simulink model "exosketon_robot_advanced_robotic"  (R2020b)
settings: Solver=FixedStepAuto  StartTime=0.0  StopTime=12  FixedStep=0.1  RelTol=1e-3
undefined symbols (not defined in the file): L_1, L_2, m_31, m_32
settings Model: Creator=A family  LastModifiedBy=A family

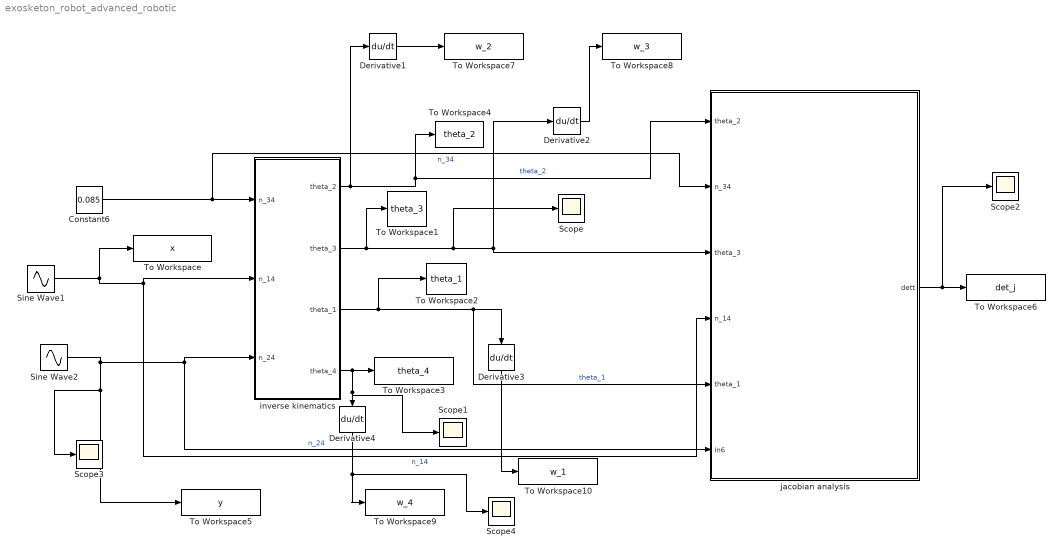
== system exosketon_robot_advanced_robotic ==
  Constant6 : Constant  Value=0.085
  Derivative{1..4} (4 alike) : Derivative
  Scope{,1..4} (5 alike) : Scope
  Sine Wave1 : Sin  Amplitude=0.2  Frequency=0.2  SampleTime=0
  Sine Wave2 : Sin  Amplitude=0.2  Frequency=0.2  Phase=-pi/2  SampleTime=0
  To Workspace : ToWorkspace  VariableName=x  SampleTime=-1
  To Workspace1 : ToWorkspace  VariableName=theta_3  SampleTime=-1
  To Workspace10 : ToWorkspace  VariableName=w_1  SampleTime=-1
  To Workspace2 : ToWorkspace  VariableName=theta_1  SampleTime=-1
  To Workspace3 : ToWorkspace  VariableName=theta_4  SampleTime=-1
  To Workspace4 : ToWorkspace  VariableName=theta_2  SampleTime=-1
  To Workspace5 : ToWorkspace  VariableName=y  SampleTime=-1
  To Workspace6 : ToWorkspace  VariableName=det_j  SampleTime=-1
  To Workspace7 : ToWorkspace  VariableName=w_2  SampleTime=-1
  To Workspace8 : ToWorkspace  VariableName=w_3  SampleTime=-1
  To Workspace9 : ToWorkspace  VariableName=w_4  SampleTime=-1
  inverse kinematics : Subsystem
  jacobian analysis : Subsystem
  wires:
  Constant6/1 -> jacobian analysis/2(n_34), inverse kinematics/1(n_34)  "n_34"
  Sine Wave1/1 -> inverse kinematics/2(n_14), jacobian analysis/4(n_14), To Workspace/1  "n_14"
  Sine Wave2/1 -> Scope3/1, To Workspace5/1, inverse kinematics/3(n_24), jacobian analysis/6(In6)  "n_24"
  inverse kinematics/4(theta_4) -> Scope1/1, Derivative4/1, To Workspace3/1
  inverse kinematics/3(theta_1) -> jacobian analysis/5(theta_1), Derivative3/1, To Workspace2/1  "theta_1"
  inverse kinematics/2(theta_3) -> Scope/1, Derivative2/1, jacobian analysis/3(theta_3), To Workspace1/1
  inverse kinematics/1(theta_2) -> Derivative1/1, To Workspace4/1, jacobian analysis/1(theta_2)  "theta_2"
  Derivative1/1 -> To Workspace7/1
  Derivative2/1 -> To Workspace8/1
  Derivative4/1 -> Scope4/1, To Workspace9/1
  Derivative3/1 -> To Workspace10/1
  jacobian analysis/1(dett) -> Scope2/1, To Workspace6/1

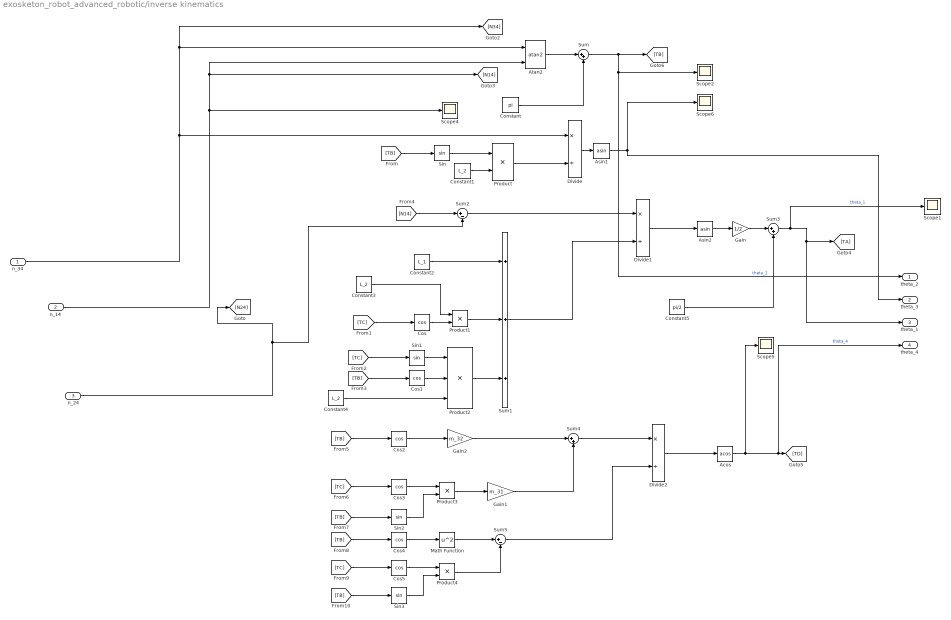
== system exosketon_robot_advanced_robotic/inverse kinematics ==
  n_34 : Inport
  n_14 : Inport  Port=2
  n_24 : Inport  Port=3
  Acos : Trigonometry  Operator=acos
  Asin1 : Trigonometry  Operator=asin
  Asin2 : Trigonometry  Operator=asin
  Atan2 : Trigonometry  Operator=atan2
  Constant : Constant  Value=pi
  Constant1 : Constant  Value=L_2
  Constant2 : Constant  Value=L_1
  Constant3 : Constant  Value=L_2
  Constant4 : Constant  Value=L_2
  Constant5 : Constant  Value=pi/2
  Cos{,1..5} (6 alike) : Trigonometry  Operator=cos
  Divide : Product  Inputs=*/
  Divide1 : Product  Inputs=*/
  Divide2 : Product  Inputs=*/
  Gain : Gain  Gain=1/2
  Gain1 : Gain  Gain=m_31
  Gain2 : Gain  Gain=m_32
  Math Function : Math  Operator=square  SaturateOnIntegerOverflow=on
  Product{,1,3..4} (4 alike) : Product
  Product2 : Product  Inputs=3
  Scope{1..2,4..6} (5 alike) : Scope
  Sin{,1..3} (4 alike) : Trigonometry
  Sum : Sum  Inputs=|++
  Sum1 : Sum  Inputs=+++
  Sum2 : Sum  Inputs=|+-
  Sum3 : Sum  Inputs=|++
  Sum4 : Sum  Inputs=|++
  Sum5 : Sum  Inputs=|+-
  theta_2 : Outport
  theta_3 : Outport  Port=2
  theta_1 : Outport  Port=3
  theta_4 : Outport  Port=4
  wires:
  Product2/1 -> Sum1/3
  Cos3/1 -> Product3/1
  Asin2/1 -> Gain/1
  Sum3/1 -> theta_1/1, [TA], Scope1/1  "theta_1"
  n_34/1 -> [N34], Atan2/1, Divide/1
  Constant1/1 -> Product/2
  Product3/1 -> Gain1/1
  Constant4/1 -> Product2/3
  Cos/1 -> Product1/2
  Asin1/1 -> theta_3/1, Scope6/1
  Constant/1 -> Sum/2
  Product/1 -> Divide/2
  Constant2/1 -> Sum1/1
  [TC] -> Cos/1
  [TB] -> Sin/1
  Sum2/1 -> Divide1/1
  Divide2/1 -> Acos/1
  [TB] -> Cos4/1
  Divide1/1 -> Asin2/1
  Product1/1 -> Sum1/2
  Sin3/1 -> Product4/2
  Constant5/1 -> Sum3/2
  Gain1/1 -> Sum4/2
  Sin/1 -> Product/1
  Sum/1 -> theta_2/1, Scope2/1, [TB]  "theta_2"
  n_24/1 -> Sum2/2, [N24]
  Atan2/1 -> Sum/1
  n_14/1 -> [N14], Atan2/2, Scope4/1
  Sin2/1 -> Product3/2
  [TB] -> Sin2/1
  [TB] -> Cos2/1
  Cos1/1 -> Product2/2
  Math Function/1 -> Sum5/1
  Sum1/1 -> Divide1/2
  Sum4/1 -> Divide2/1
  Sum5/1 -> Divide2/2
  Gain2/1 -> Sum4/1
  Divide/1 -> Asin1/1
  Gain/1 -> Sum3/1
  Cos2/1 -> Gain2/1
  [TB] -> Cos1/1
  Acos/1 -> theta_4/1, [TD], Scope5/1  "theta_4"
  Sin1/1 -> Product2/1
  [TC] -> Sin1/1
  Constant3/1 -> Product1/1
  [TC] -> Cos5/1
  Cos4/1 -> Math Function/1
  [TB] -> Sin3/1
  Cos5/1 -> Product4/1
  Product4/1 -> Sum5/2
  [TC] -> Cos3/1
  [N14] -> Sum2/1

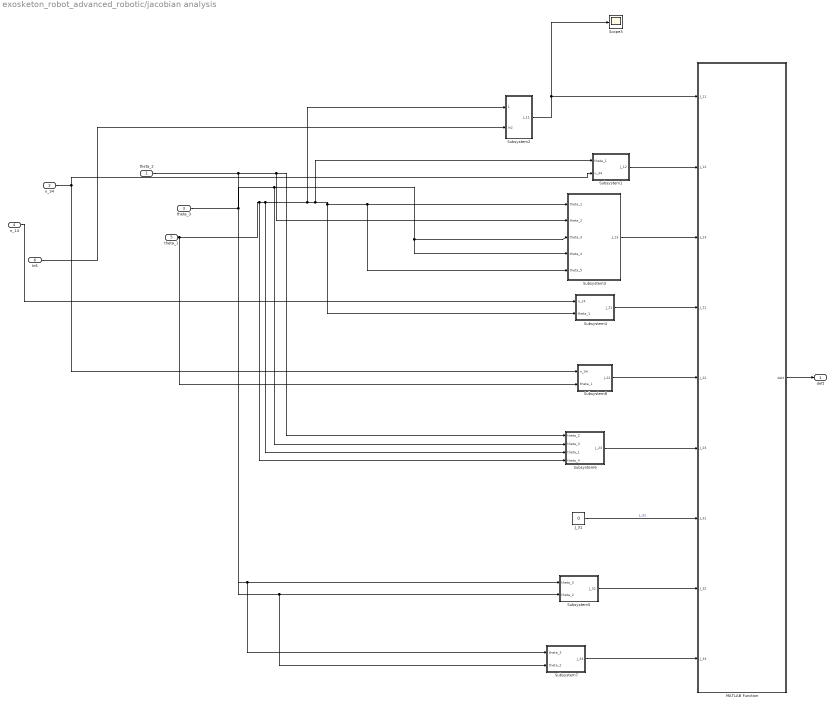
== system exosketon_robot_advanced_robotic/jacobian analysis ==
  theta_2 : Inport
  n_34 : Inport  Port=2
  theta_3 : Inport  Port=3
  n_14 : Inport  Port=4
  theta_1 : Inport  Port=5
  In6 : Inport  Port=6
  J_31 : Constant  Value=0
  MATLAB Function : MATLAB Function  TreatAsAtomicUnit=on
  Scope3 : Scope
  Subsystem1 : Subsystem
  Subsystem2 : Subsystem
  Subsystem3 : Subsystem
  Subsystem4 : Subsystem
  Subsystem5 : Subsystem
  Subsystem6 : Subsystem
  Subsystem7 : Subsystem
  Subsystem8 : Subsystem
  dett : Outport
  wires:
  Subsystem6/1(J_23) -> MATLAB Function/6(J_23)
  n_34/1 -> Subsystem8/1(n_34), Subsystem1/2(n_34)
  Subsystem5/1(J_32) -> MATLAB Function/8(J_32)
  Subsystem1/1(J_12) -> MATLAB Function/2(J_12)
  theta_1/1 -> Subsystem3/5(theta_5), Subsystem3/1(theta_1), Subsystem4/2(theta_1), Subsystem1/1(theta_1), Subsystem2/1(theta_1), Subsystem6/3(theta_1), Subsystem6/4(theta_4), Subsystem8/2(theta_1)
  theta_2/1 -> Subsystem6/1(theta_2), Subsystem3/2(theta_2), Subsystem7/2(theta_2), Subsystem5/2(theta_2)
  Subsystem2/1(J_11) -> Scope3/1, MATLAB Function/1(J_11)
  J_31/1 -> MATLAB Function/7(J_31)  "J_31"
  Subsystem4/1(J_21) -> MATLAB Function/4(J_21)
  theta_3/1 -> Subsystem6/2(theta_3), Subsystem3/4(theta_4), Subsystem3/3(theta_3), Subsystem7/1(theta_3), Subsystem5/1(theta_3)
  Subsystem8/1(J-22) -> MATLAB Function/5(J_22)
  Subsystem7/1(J_33) -> MATLAB Function/9(J_33)
  Subsystem3/1(J_13) -> MATLAB Function/3(J_13)
  MATLAB Function/1(dett) -> dett/1
  n_14/1 -> Subsystem4/1(n_14)
  In6/1 -> Subsystem2/2(In2)

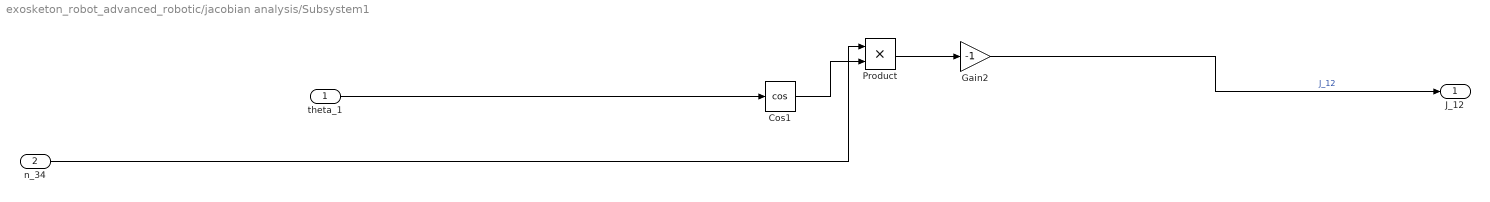
== system exosketon_robot_advanced_robotic/jacobian analysis/Subsystem1 ==
  theta_1 : Inport
  n_34 : Inport  Port=2
  Cos1 : Trigonometry  Operator=cos
  Gain2 : Gain  Gain=-1
  Product : Product
  J_12 : Outport
  wires:
  n_34/1 -> Product/1
  Product/1 -> Gain2/1
  Cos1/1 -> Product/2
  theta_1/1 -> Cos1/1
  Gain2/1 -> J_12/1  "J_12"

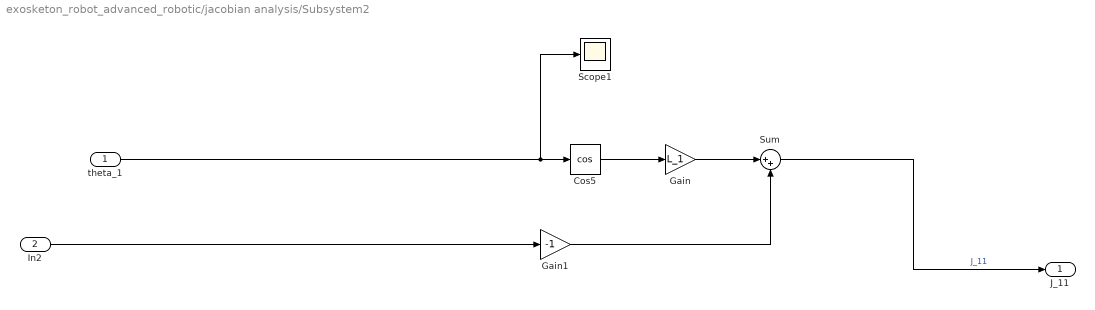
== system exosketon_robot_advanced_robotic/jacobian analysis/Subsystem2 ==
  theta_1 : Inport
  In2 : Inport  Port=2
  Cos5 : Trigonometry  Operator=cos
  Gain : Gain  Gain=L_1
  Gain1 : Gain  Gain=-1
  Scope1 : Scope
  Sum : Sum  Inputs=|++
  J_11 : Outport
  wires:
  Cos5/1 -> Gain/1
  In2/1 -> Gain1/1
  Sum/1 -> J_11/1  "J_11"
  Gain1/1 -> Sum/2
  theta_1/1 -> Scope1/1, Cos5/1
  Gain/1 -> Sum/1

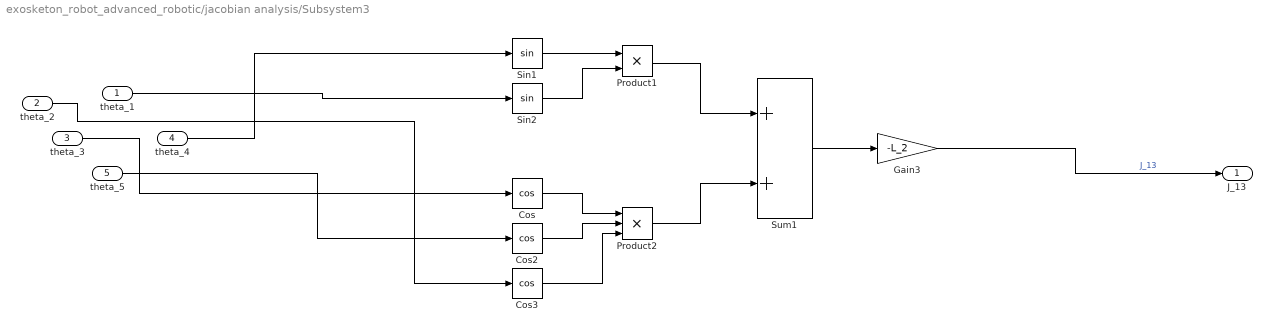
== system exosketon_robot_advanced_robotic/jacobian analysis/Subsystem3 ==
  theta_1 : Inport
  theta_2 : Inport  Port=2
  theta_3 : Inport  Port=3
  theta_4 : Inport  Port=4
  theta_5 : Inport  Port=5
  Cos : Trigonometry  Operator=cos
  Cos2 : Trigonometry  Operator=cos
  Cos3 : Trigonometry  Operator=cos
  Gain3 : Gain  Gain=-L_2
  Product1 : Product
  Product2 : Product  Inputs=3
  Sin1 : Trigonometry
  Sin2 : Trigonometry
  Sum1 : Sum
  J_13 : Outport
  wires:
  Sin2/1 -> Product1/2
  Product2/1 -> Sum1/2
  Cos/1 -> Product2/1
  theta_3/1 -> Cos/1
  Sin1/1 -> Product1/1
  theta_4/1 -> Sin1/1
  Product1/1 -> Sum1/1
  Cos3/1 -> Product2/3
  theta_1/1 -> Sin2/1
  Cos2/1 -> Product2/2
  Sum1/1 -> Gain3/1
  theta_2/1 -> Cos3/1
  Gain3/1 -> J_13/1  "J_13"
  theta_5/1 -> Cos2/1

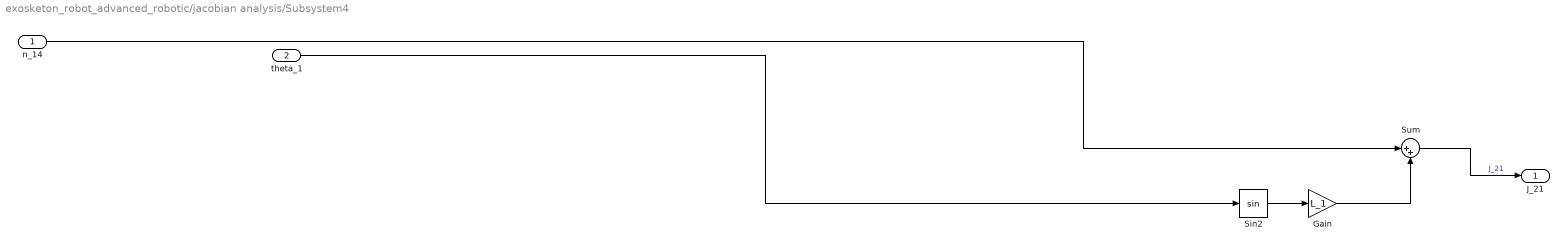
== system exosketon_robot_advanced_robotic/jacobian analysis/Subsystem4 ==
  n_14 : Inport
  theta_1 : Inport  Port=2
  Gain : Gain  Gain=L_1
  Sin2 : Trigonometry
  Sum : Sum  Inputs=|++
  J_21 : Outport
  wires:
  Gain/1 -> Sum/2
  Sin2/1 -> Gain/1
  n_14/1 -> Sum/1
  theta_1/1 -> Sin2/1
  Sum/1 -> J_21/1  "J_21"

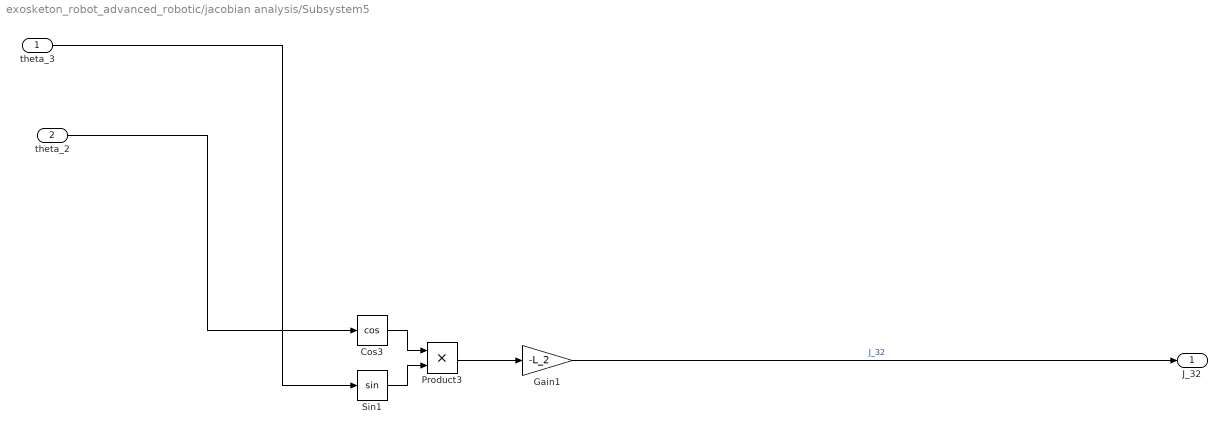
== system exosketon_robot_advanced_robotic/jacobian analysis/Subsystem5 ==
  theta_3 : Inport
  theta_2 : Inport  Port=2
  Cos3 : Trigonometry  Operator=cos
  Gain1 : Gain  Gain=-L_2
  Product3 : Product
  Sin1 : Trigonometry
  J_32 : Outport
  wires:
  Gain1/1 -> J_32/1  "J_32"
  theta_2/1 -> Cos3/1
  Cos3/1 -> Product3/1
  Sin1/1 -> Product3/2
  Product3/1 -> Gain1/1
  theta_3/1 -> Sin1/1

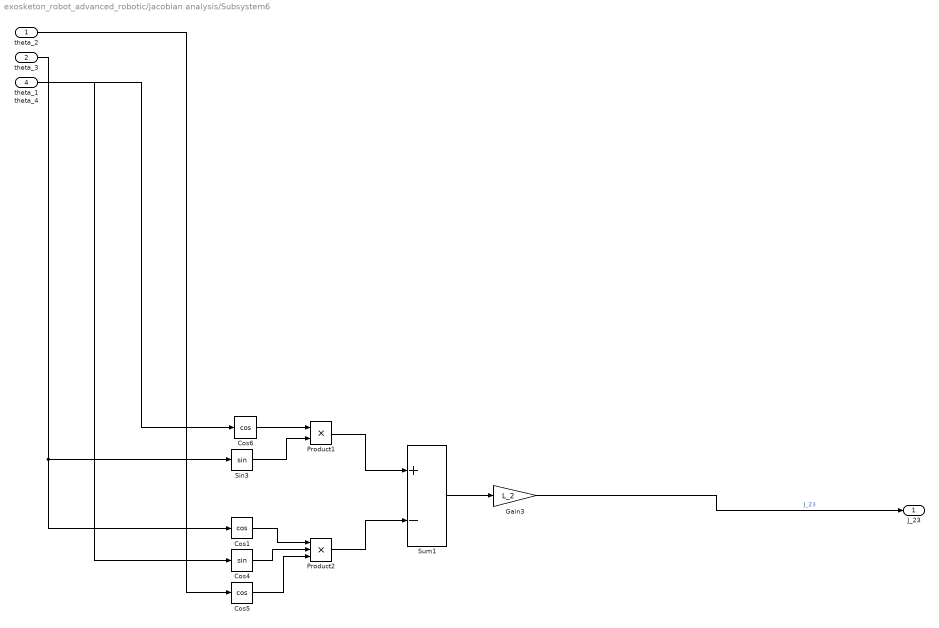
== system exosketon_robot_advanced_robotic/jacobian analysis/Subsystem6 ==
  theta_2 : Inport
  theta_3 : Inport  Port=2
  theta_1 : Inport  Port=3
  theta_4 : Inport  Port=4
  Cos1 : Trigonometry  Operator=cos
  Cos4 : Trigonometry
  Cos5 : Trigonometry  Operator=cos
  Cos6 : Trigonometry  Operator=cos
  Gain3 : Gain  Gain=L_2
  Product1 : Product
  Product2 : Product  Inputs=3
  Sin3 : Trigonometry
  Sum1 : Sum  Inputs=+-
  J_23 : Outport
  wires:
  Cos5/1 -> Product2/3
  Cos1/1 -> Product2/1
  theta_3/1 -> Cos1/1, Sin3/1
  Cos4/1 -> Product2/2
  Product1/1 -> Sum1/1
  Sum1/1 -> Gain3/1
  Sin3/1 -> Product1/2
  Cos6/1 -> Product1/1
  theta_2/1 -> Cos5/1
  Product2/1 -> Sum1/2
  Gain3/1 -> J_23/1  "J_23"
  theta_4/1 -> Cos6/1
  theta_1/1 -> Cos4/1

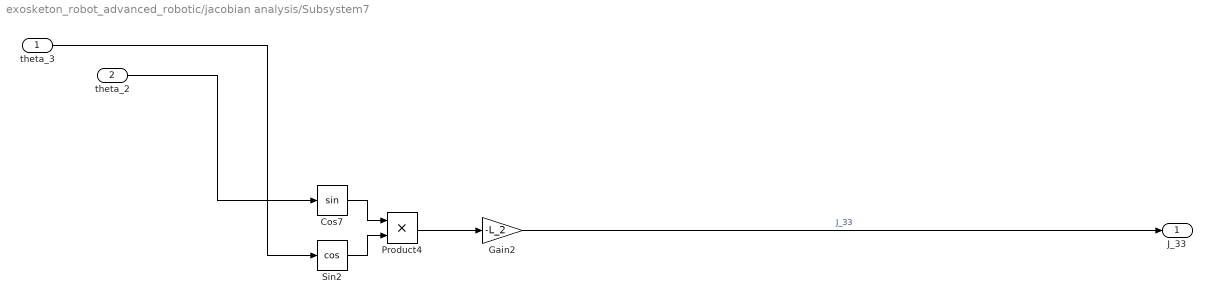
== system exosketon_robot_advanced_robotic/jacobian analysis/Subsystem7 ==
  theta_3 : Inport
  theta_2 : Inport  Port=2
  Cos7 : Trigonometry
  Gain2 : Gain  Gain=-L_2
  Product4 : Product
  Sin2 : Trigonometry  Operator=cos
  J_33 : Outport
  wires:
  Product4/1 -> Gain2/1
  Cos7/1 -> Product4/1
  Sin2/1 -> Product4/2
  theta_2/1 -> Cos7/1
  theta_3/1 -> Sin2/1
  Gain2/1 -> J_33/1  "J_33"

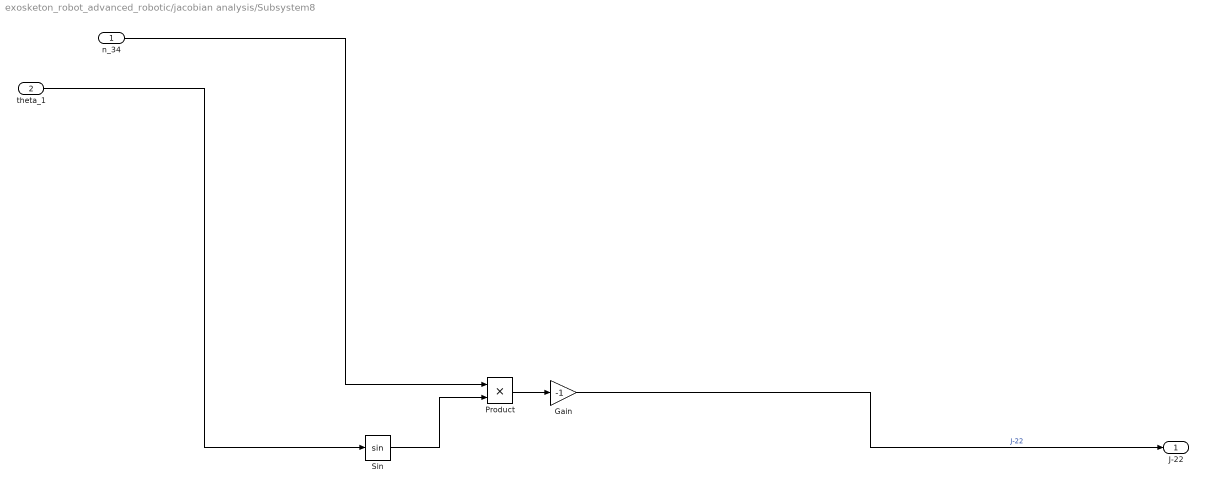
== system exosketon_robot_advanced_robotic/jacobian analysis/Subsystem8 ==
  n_34 : Inport
  theta_1 : Inport  Port=2
  Gain : Gain  Gain=-1
  Product : Product
  Sin : Trigonometry
  J-22 : Outport
  wires:
  Sin/1 -> Product/2
  Product/1 -> Gain/1
  Gain/1 -> J-22/1  "J-22"
  n_34/1 -> Product/1
  theta_1/1 -> Sin/1

== matlab function exosketon_robot_advanced_robotic/jacobian analysis/MATLAB Function ==
  data: J_11 input; dett output; J_12 input; J_13 input; J_21 input; J_22 input; J_23 input; J_31 input; J_32 input; J_33 input
function dett = jacobe(J_11, J_12, J_13, J_21, J_22, J_23, J_31, J_32, J_33)

dett = J_11*J_22*J_33 - J_11*J_23*J_32 - J_12*J_21*J_33 + J_13*J_21*J_32
